simulink model "cvtModel_dashboard_mapped"  (R2023a)
settings: Solver=VariableStepAuto  StartTime=0.0  StopTime=inf  FixedStep=1e-3  RelTol=1e-3  AbsTol=1e-3  EnableMultiTasking=on
PreLoadFcn:
  | m1=3.5;
  | m2=3.2;
  | mr1=0.8;
  | mr2=0.7;
  | speedVector=[1508.85099817596;1518.45723596462;1530.44196592720;1537.65262467286;1544.87011816615;1563.98348990289;1583.08660951818;1616.48460379372;1668.91395283447;1709.42350201510;1752.30812599583;1799.96340381967;1847.59134265301;1904.74008492967;1971.45405650923;2028.61646828115;2083.40038787914;2140.55254752961;2190.54189166781;2259.62068592604;2323.95274795787;2376.37867962481;2443.06531221387;2519.28983511532;2576.50350749443;2612.24923757958;2650.37004246484;2681.37245769738;2717.13869202541;2771.92602899721;2819.56080257817;2855.26894155137;2890.95315890788;2938.61868885316;2976.76341535511;2991.07537688442;3019.63778721441;3045.79436637996;3071.94069342408;3093.34370561560;3114.80823053575;3141.04340929901;3172.04240715774;3186.35436868705;3214.89627477416;3231.51496362732;3267.18209411476;3333.83797033950;3371.93485360807;3421.93444986770;3488.60057821388;3540.98550139507;3586.19052219491;3617.10408570831;3674.22548899447;3712.24719003915;3731.22044944954;3740.69340965949;3759.66325169607;3771.50786933232;3785.72414439486;3792.79810818800;3797.48674505959;3802.17879930499;3806.87085355039;3816.26521416264;3820.89917305322;3827.93896310823;3835.00950952755;3839.71865064202];
  | torqueVector=[15.4893802008608;16.0795925394548;16.6441434720229;17.1317101865136;17.6705997130559;18.1068436154950;18.4661032998565;18.8510243902439;19.0563156384505;19.1846226685796;19.2616068866571;19.3899139167862;19.3129296987087;19.1846226685796;19.3385911047346;19.3129296987087;19.3129296987087;19.2102840746054;18.9793314203730;19.0049928263988;19.1589612625538;19.3385911047346;19.2872682926829;19.3129296987087;19.6721893830703;19.8004964131994;19.8774806312769;20.1597560975610;20.4420315638450;20.4676929698709;20.4420315638450;20.2880631276901;19.9544648493544;20.1597560975610;20.4163701578192;20.5703385939742;20.4163701578192;20.0827718794835;19.6721893830703;19.4155753228120;19.6208665710186;19.8774806312769;20.1340946915351;20.2880631276901;19.9801262553802;19.5695437589670;19.1076384505021;18.8253629842181;18.7227173601148;18.5687489239598;18.3634576757532;18.2351506456241;17.8502295552367;17.4653084648493;17.1317101865136;16.4645136298422;15.8486398852224;15.4380573888092;14.7965222381636;14.3089555236729;13.7444045911047;13.2055150645624;12.6409641319943;12.1020746054519;11.5631850789096;10.5623902439024;9.58725681492108;8.79175322812051;8.22720229555236;7.81661979913916];
  | load Lookuptable_data
model workspace (MAT data in the model file):
  DOWN_TABLE = [0  5  20  35; 0  5  20  35; 0  5  25  40; 0  5  30  50; 0  30  50  80; 0  30  50  80]
  DOWN_TH_BP = [0; 0.05; 0.4; 0.5; 0.9; 1]
  TWAIT = 2
  UP_TABLE = [10  30  50  1000000; 10  30  50  1000000; 15  30  50  1000000; 23  41  60  1000000; 40  70  100  1000000; 40  70  100  1000000]
  UP_TH_BP = [0; 0.25; 0.35; 0.5; 0.9; 1]
  clutchRise = 0.1
  eff_tor_rad = 0.4
  engagement_area = 0.0025
  fric_coeff = 0.5
  num_fric_surf = 6
  p0 = 2000000
  peak_normal = 0.55
  pressThresh = 0.05
  velTol = 0.001
undefined symbols (not defined in the file): vehicle_speed
libraries: fl_lib x22, sdl_lib x9, nesl_utility x8
(part 1 of 2)
CloseFcn:
  | try,close(h1_sdl_car),end
  | clear h1_sdl_car
  | 
  | clear simlog_sdl_car
  | clear logsout_sdl_car
Description:
  | Vehicle with Four-Speed Transmission
  | 
  | Copyright 2008-2016 The MathWorks, Inc.
settings Model: PacingRate=5  Creator=MathWorks
settings SolverCC: AutoScaleAbsTol=off  ZcThreshold=0  ZeroCrossAlgorithm=Adaptive  AlgebraicLoopSolver=TrustRegion
settings DataIOCC: LimitDataPoints=on  MaxDataPoints=10000  SaveOutput=off  DSMLogging=off  SaveTime=off  ReturnWorkspaceOutputs=off  SignalLoggingName=logsout_cvtModel_dashboard
settings OptimizationCC: ExpressionDepthLimit=2147483647  InitFltsAndDblsToZero=on  LifeSpan=inf
settings DebuggingCC: AlgebraicLoopMsg=none  SaveWithParameterizedLinksMsg=none  UnderspecifiedInitializationDetection=Classic  MergeDetectMultiDrivingBlocksExec=none  CheckExecutionContextPreStartOutputMsg=on  SignalResolutionControl=TryResolveAllWithWarning  MaskedZcDiagnostic=none  MultiTaskDSMMsg=warning  MultiTaskCondExecSysMsg=none  SigSpecEnsureSampleTimeMsg=none  FcnCallInpInsideContextMsg=warning  UnconnectedInputMsg=warning  UnconnectedOutputMsg=warning  UnconnectedLineMsg=warning  AllowSymbolicDim=off  StateNameClashWarn=warning  SFUnexpectedBacktrackingDiag=warning  SFNoUnconditionalDefaultTransitionDiag=warning  SFExecutionAtInitializationDiag=none  ArithmeticOperatorsInVariantConditions=warning
settings HardwareCC: ProdBitPerPointer=32  ProdBitPerSizeT=32  ProdBitPerPtrDiffT=32  ProdLargestAtomicFloat=None  ProdIntDivRoundTo=Undefined  ProdEndianess=Unspecified  ProdWordSize=32  ProdHWDeviceType=32-bit Generic  TargetBitPerLong=64  TargetBitPerPointer=64  TargetBitPerSizeT=64  TargetBitPerPtrDiffT=64  TargetLongLongMode=on  TargetIntDivRoundTo=Zero  TargetEndianess=LittleEndian  TargetWordSize=64  TargetHWDeviceType=MATLAB Host  ProdEqTarget=off
settings ModelReferenceCC: UpdateModelReferenceTargets=IfOutOfDate  EnableRefExpFcnMdlSchedulingChecks=on  PropagateSignalLabelsOutOfModel=off
settings SFSimCC: SimUseLocalCustomCode=off  CustomCodeUndefinedFunction=UseInterfaceOnly
settings RTWCC: RTWUseLocalCustomCode=off
settings CodeAppCC: StateflowObjectComments=on
settings GRTTargetCC: TargetLangStandard=C89/C90 (ANSI)  CombineOutputUpdateFcns=off  GRTInterface=on
settings ConfigComp: CovMetricSettings=dw  CovSaveCumulativeToWorkspaceVar=on  CovSaveSingleToWorkspaceVar=on  CovExternalEMLEnable=off  CovBoundaryAbsTol=1.0e-5
settings SimscapeCC: SimscapeNormalizeSystem=off  SimscapeLogType=all  SimscapeLogSimulationStatistics=on

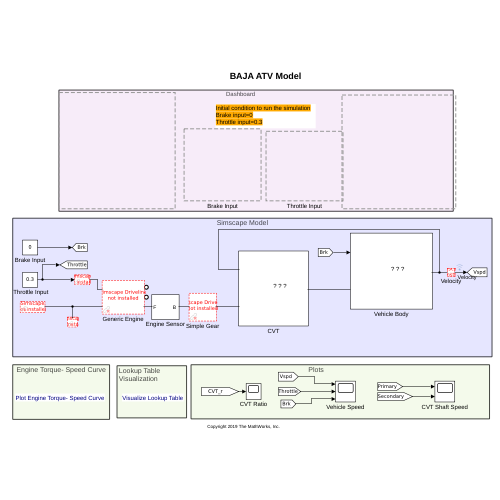
[thumbnail: Simulink's stored preview of the top-level diagram]
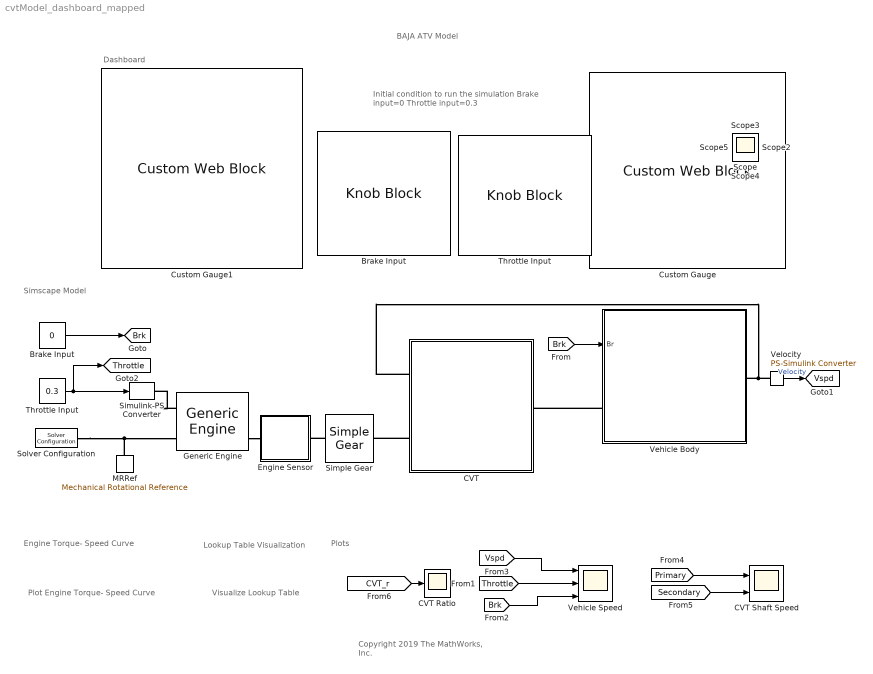
== system cvtModel_dashboard_mapped ==
  note: Initial condition to run the simulation
      | Brake input=0
      | Throttle input=0.3
  note: Dashboard
  note: Simscape Model
  note: Copyright 2019 The MathWorks, Inc.
  note: Plots
  note: Visualize Lookup Table
  note: Lookup Table
      | Visualization
  note: Engine Torque- Speed Curve
  note: Plot Engine Torque- Speed Curve
  note: BAJA ATV Model
  "   Throttle Input " : Constant  Value=0.3
  Brake Input : KnobBlock  LabelPosition=Hide  ScaleMax=0.5  TickInterval=0.10000000000000001
  "Brake Input " : Constant  Value=0
  CVT : Subsystem
      mask Display: image("CVT.jpg")
  CVT Ratio : Scope
  CVT Shaft Speed : Scope  NumInputPorts=2
  Custom Gauge : CustomWebBlock  LabelPosition=Bottom  ShowInitialText=on  Configuration="{\"components\":[{\"name\":\"CircularScaleComponent\",\"settings\":{\"bounds\":{\"max\":100,\"min\":0,\"tickInterval\":\"auto\"},\"direction\":\"cw\",\"flipLimits\":0,\"innerRadius\":0.75,\"internalTickHeightScaleFactor\":1,\"labelColor\":[255,252,199],\"labelFont\":{\"font\":\"Arial\",\"fontSize\":12},\"labelRadius\":0.36,\"labelTransparency\":1,\"minorTickHeightScaleFactor\":0.2,\"needleImage\":{\"size\":[1890,567],\"src\":\"data:image\\/svg+xml;base64,PD94bWwgdmVyc2lvbj0iMS4wIiBlbmNvZGluZz0iVVRGLTgiIHN0YW5kYWxvbmU9Im5vIj8+CjxzdmcKICAgeG1sbnM6ZGM9Imh0dHA6Ly9wdXJsLm9yZy9kYy9lbGVtZW50cy8xLjEvIgogICB4bWxuczpjYz0iaHR0cDovL2NyZWF0aXZlY29tbW9ucy5vcmcvbnMjIgogICB4bWxuczpyZGY9Imh0dHA6Ly93d3cudzMub3JnLzE5OTkvMDIvMjItcmRmLXN5bnRheC1ucyMiCiAgIHhtbG5zOnN2Zz0iaHR0cDovL3d3dy53My5vcmcvMjAwMC9zdmciCiAgIHhtbG5zPSJodHRwOi8vd3d3LnczLm9yZy8yMDAwL3N2ZyIKICAgeG1sbnM6 ...(+4096 chars)\"},\"needleOffset\":[0.14,0],\"needleOrientation\":-45,\"needleRotation\":180,\"needleSize\":{\"height\":0.13,\"width\":0.41},\"outerRadius\":0.9,\"position\":[0.06486742424242424,0.05627705627705628,0.8917748917748918,0.8787878787878788],\"scaleAngle\":270,\"scaleAngleOffset\":135,\"scaleColors\":[],\"scaleColorsSize\":0.2,\"scalePosition\":[0,0,1,1],\"showLabels\":1,\"showMinorTicks\":1,\"showSpanLine\":1,\"showTicks\":1,\"tickColor\":[255,255,200],\"tickTransparency\":1,\"valueBarColor\":[0,114,189],\"valueBarPosition\":[0,0,1,1],\"valueBarSize\":0.2,\"valueBarTransparency\":1}},{\"name\":\"BackgroundImageComponent\",\"settings\":{\"image\":{\"size\":[500,500],\"src\":\"data:image\\/svg+xml;base64,PD94bWwgdmVyc2lvbj0iMS4wIiBlbmNvZGluZz0iVVRGLTgiIHN0YW5kYWxvbmU9Im5vIj8+CjxzdmcKICAgeG1sbnM6ZGM9Imh0dHA6Ly9wdXJsLm9yZy9kYy9lbGVtZW50cy8xLjEvIgogICB4bWxuczpjYz0iaHR0cDovL2NyZWF0aXZlY29tbW9ucy5vcmcvbnMjIgogICB4bWxuczpyZGY9Imh0dHA6Ly93d3cudzMub3JnLzE5OTkvMDIvMjItcmRmLXN5bnRheC1ucyMiCiAgIHhtbG5zOnN2Zz0iaHR0cDovL3d3dy53My5vcmcvMjAwMC9zdmciCiAgIHhtbG5zPSJodHRwOi8vd3d3LnczLm9yZy8yMDAwL3N2ZyIKICAgeG1sbnM6 ...(+9964 chars)\"},\"position\":[0,0,1,1],\"scaleMode\":\"0\"}},{\"name\":\"ForegroundImageComponent\",\"settings\":{\"image\":{\"size\":[0,0],\"src\":\"default\",\"srcOrientation\":[]},\"isForeground\":1,\"position\":[0,0,1,1],\"scaleMode\":\"0\"}}],\"legacySettings\":{\"BackgroundImage\":\"data:image\\/svg+xml;base64,PD94bWwgdmVyc2lvbj0iMS4wIiBlbmNvZGluZz0iVVRGLTgiIHN0YW5kYWxvbmU9Im5vIj8+CjwhLS0gR2VuZXJhdG9yOiBBZG9iZSBJbGx1c3RyYXRvciAxOS4yLjEsIFNWRyBFeHBvcnQgUGx1Zy1JbiAuIFNWRyBWZXJzaW9uOiA2LjAwIEJ1aWxkIDApICAtLT4KCjxzdmcKICAgeG1sbnM6ZGM9Imh0dHA6Ly9wdXJsLm9yZy9kYy9lbGVtZW50cy8xLjEvIgogICB4bWxuczpjYz0iaHR0cDovL2NyZWF0aXZlY29tbW9ucy5vcmcvbnMjIgogICB4bWxuczpyZGY9Imh0dHA6Ly93d3cudzMub3JnLzE5OTkvMDIvMjItcmRmLXN5bnRh ...(+9660 chars)\",\"CenterOffsetX\":\"0\",\"CenterOffsetY\":\"0\",\"GaugeArcColor\":\"#9ec0f7\",\"GaugeArcDefined\":\"true\",\"GaugeArcRadius\":\"0.1358563990074277\",\"GaugeArcRatio\":\"0.8333333333333\",\"GaugeArcRotation\":\"240.5385250290321\",\"GaugeArcStrokeWidth\":\"0.03972965542329953\",\"GaugeArcTransparency\":\"0\",\"GaugeMax\":\"100\",\"GaugeMin\":\"0\",\"GaugeTickColor\":\"#faf5c8\",\"GaugeTickTransparency\":\"1\",\"GaugeTickVisible\":\"true\",\"GaugeValue\":\"0\",\"NeedleHeight\":\"0.11602152693163792\",\"NeedleImage\":\"data:image\\/svg+xml;base64,PD94bWwgdmVyc2lvbj0iMS4wIiBlbmNvZGluZz0idXRmLTgiPz4KPCEtLSBHZW5lcmF0b3I6IEFkb2JlIElsbHVzdHJhdG9yIDE5LjIuMSwgU1ZHIEV4cG9ydCBQbHVnLUluIC4gU1ZHIFZlcnNpb246IDYuMDAgQnVpbGQgMCkgIC0tPgo8c3ZnIHZlcnNpb249IjEuMSIgeG1sbnM9Imh0dHA6Ly93d3cudzMub3JnLzIwMDAvc3ZnIiB4bWxuczp4bGluaz0iaHR0cDovL3d3dy53My5vcmcvMTk5OS94bGluayIgeD0iMHB4IiB5PSIwcHgiCgkgdmlld0JveD0iMCAwIDIwMCA1MCIgc3R5bGU9ImVuYWJsZS1iYWNrZ3JvdW5kOm5ldyAw ...(+9940 chars)\",\"NeedleInitialRotation\":\"-59.94322499147643\",\"NeedleWidth\":\"0.1911368983686954\",\"NeedleXPos\":\"0.3802298124325669\",\"NeedleYPos\":\"0.48117305677424654\",\"ScaleColorsJSON\":\"{\\\"Min\\\":0,\\\"Max\\\":0,\\\"Color\\\":[0,0.44705882352941173,0.74117647058823533]}\",\"ValueArcColor\":\"#1759b0\",\"ValueArcTransparency\":\"1\"},\"settings\":{\"BindingType\":\"signal\",\"backgroundOffset\":0.14,\"backgroundOpacity\":1,\"fixedAspectRatio\":\"on\",\"showBackgroundColor\":0,\"version\":\"R2023a\"},\"type\":\"CircularGauge\"}"
  Custom Gauge1 : CustomWebBlock  LabelPosition=Bottom  ShowInitialText=on  Configuration="{\"components\":[{\"name\":\"CircularScaleComponent\",\"settings\":{\"bounds\":{\"max\":100,\"min\":0,\"tickInterval\":\"auto\"},\"direction\":\"cw\",\"flipLimits\":0,\"innerRadius\":0.75,\"internalTickHeightScaleFactor\":1,\"labelColor\":[255,252,199],\"labelFont\":{\"font\":\"Arial\",\"fontSize\":12},\"labelRadius\":0.36,\"labelTransparency\":1,\"minorTickHeightScaleFactor\":0.2,\"needleImage\":{\"size\":[1890,567],\"src\":\"data:image\\/svg+xml;base64,PD94bWwgdmVyc2lvbj0iMS4wIiBlbmNvZGluZz0iVVRGLTgiIHN0YW5kYWxvbmU9Im5vIj8+CjxzdmcKICAgeG1sbnM6ZGM9Imh0dHA6Ly9wdXJsLm9yZy9kYy9lbGVtZW50cy8xLjEvIgogICB4bWxuczpjYz0iaHR0cDovL2NyZWF0aXZlY29tbW9ucy5vcmcvbnMjIgogICB4bWxuczpyZGY9Imh0dHA6Ly93d3cudzMub3JnLzE5OTkvMDIvMjItcmRmLXN5bnRheC1ucyMiCiAgIHhtbG5zOnN2Zz0iaHR0cDovL3d3dy53My5vcmcvMjAwMC9zdmciCiAgIHhtbG5zPSJodHRwOi8vd3d3LnczLm9yZy8yMDAwL3N2ZyIKICAgeG1sbnM6 ...(+4096 chars)\"},\"needleOffset\":[0.14,0],\"needleOrientation\":-45,\"needleRotation\":180,\"needleSize\":{\"height\":0.13,\"width\":0.41},\"outerRadius\":0.9,\"position\":[0.06486742424242424,0.05627705627705628,0.8917748917748918,0.8787878787878788],\"scaleAngle\":270,\"scaleAngleOffset\":135,\"scaleColors\":[],\"scaleColorsSize\":0.2,\"scalePosition\":[0,0,1,1],\"showLabels\":1,\"showMinorTicks\":1,\"showSpanLine\":1,\"showTicks\":1,\"tickColor\":[255,255,200],\"tickTransparency\":1,\"valueBarColor\":[0,114,189],\"valueBarPosition\":[0,0,1,1],\"valueBarSize\":0.2,\"valueBarTransparency\":1}},{\"name\":\"BackgroundImageComponent\",\"settings\":{\"image\":{\"size\":[500,500],\"src\":\"data:image\\/svg+xml;base64,PD94bWwgdmVyc2lvbj0iMS4wIiBlbmNvZGluZz0iVVRGLTgiIHN0YW5kYWxvbmU9Im5vIj8+CjxzdmcKICAgeG1sbnM6ZGM9Imh0dHA6Ly9wdXJsLm9yZy9kYy9lbGVtZW50cy8xLjEvIgogICB4bWxuczpjYz0iaHR0cDovL2NyZWF0aXZlY29tbW9ucy5vcmcvbnMjIgogICB4bWxuczpyZGY9Imh0dHA6Ly93d3cudzMub3JnLzE5OTkvMDIvMjItcmRmLXN5bnRheC1ucyMiCiAgIHhtbG5zOnN2Zz0iaHR0cDovL3d3dy53My5vcmcvMjAwMC9zdmciCiAgIHhtbG5zPSJodHRwOi8vd3d3LnczLm9yZy8yMDAwL3N2ZyIKICAgeG1sbnM6 ...(+9964 chars)\"},\"position\":[0,0,1,1],\"scaleMode\":\"0\"}},{\"name\":\"ForegroundImageComponent\",\"settings\":{\"image\":{\"size\":[0,0],\"src\":\"default\",\"srcOrientation\":[]},\"isForeground\":1,\"position\":[0,0,1,1],\"scaleMode\":\"0\"}}],\"legacySettings\":{\"BackgroundImage\":\"data:image\\/svg+xml;base64,PD94bWwgdmVyc2lvbj0iMS4wIiBlbmNvZGluZz0iVVRGLTgiIHN0YW5kYWxvbmU9Im5vIj8+CjwhLS0gR2VuZXJhdG9yOiBBZG9iZSBJbGx1c3RyYXRvciAxOS4yLjEsIFNWRyBFeHBvcnQgUGx1Zy1JbiAuIFNWRyBWZXJzaW9uOiA2LjAwIEJ1aWxkIDApICAtLT4KCjxzdmcKICAgeG1sbnM6ZGM9Imh0dHA6Ly9wdXJsLm9yZy9kYy9lbGVtZW50cy8xLjEvIgogICB4bWxuczpjYz0iaHR0cDovL2NyZWF0aXZlY29tbW9ucy5vcmcvbnMjIgogICB4bWxuczpyZGY9Imh0dHA6Ly93d3cudzMub3JnLzE5OTkvMDIvMjItcmRmLXN5bnRh ...(+9660 chars)\",\"CenterOffsetX\":\"0\",\"CenterOffsetY\":\"0\",\"GaugeArcColor\":\"#9ec0f7\",\"GaugeArcDefined\":\"true\",\"GaugeArcRadius\":\"0.1358563990074277\",\"GaugeArcRatio\":\"0.8333333333333\",\"GaugeArcRotation\":\"240.5385250290321\",\"GaugeArcStrokeWidth\":\"0.03972965542329953\",\"GaugeArcTransparency\":\"0\",\"GaugeMax\":\"10000\",\"GaugeMin\":\"0\",\"GaugeTickColor\":\"#faf5c8\",\"GaugeTickTransparency\":\"1\",\"GaugeTickVisible\":\"true\",\"GaugeValue\":\"0\",\"NeedleHeight\":\"0.11602152693163792\",\"NeedleImage\":\"data:image\\/svg+xml;base64,PD94bWwgdmVyc2lvbj0iMS4wIiBlbmNvZGluZz0idXRmLTgiPz4KPCEtLSBHZW5lcmF0b3I6IEFkb2JlIElsbHVzdHJhdG9yIDE5LjIuMSwgU1ZHIEV4cG9ydCBQbHVnLUluIC4gU1ZHIFZlcnNpb246IDYuMDAgQnVpbGQgMCkgIC0tPgo8c3ZnIHZlcnNpb249IjEuMSIgeG1sbnM9Imh0dHA6Ly93d3cudzMub3JnLzIwMDAvc3ZnIiB4bWxuczp4bGluaz0iaHR0cDovL3d3dy53My5vcmcvMTk5OS94bGluayIgeD0iMHB4IiB5PSIwcHgiCgkgdmlld0JveD0iMCAwIDIwMCA1MCIgc3R5bGU9ImVuYWJsZS1iYWNrZ3JvdW5kOm5ldyAw ...(+9940 chars)\",\"NeedleInitialRotation\":\"-59.94322499147643\",\"NeedleWidth\":\"0.1911368983686954\",\"NeedleXPos\":\"0.3802298124325669\",\"NeedleYPos\":\"0.48117305677424654\",\"ScaleColorsJSON\":\"{\\\"Min\\\":0,\\\"Max\\\":0,\\\"Color\\\":[0.92941176470588238,0.69411764705882351,0.12549019607843137]}\",\"ValueArcColor\":\"#1759b0\",\"ValueArcTransparency\":\"1\"},\"settings\":{\"BindingType\":\"signal\",\"backgroundOffset\":0.14,\"backgroundOpacity\":1,\"fixedAspectRatio\":\"on\",\"showBackgroundColor\":0,\"version\":\"R2023a\"},\"type\":\"CircularGauge\"}"
  Engine Sensor : Subsystem
  Generic Engine : sdl_lib/Engines/Generic Engine  model_parameterization=2  engine_type=1  P_max=100 kW  w_P_max=4500 rpm  w_max=5000 rpm  w_min=500 rpm  w_tab=speedVector rpm  trq_tab=torqueVector N*m  pwr_tab=[20, 40, 78, 120, 145, 148, 125, 60] kW  interp_method=simscape.enum.interpolation.linear  model_inertia=1  inertia=1 kg*m^2  initial_velocity=2100 rpm  model_time_constant=0  time_constant=0.4 s  T0=0  w_thr=100 rpm  idle_speed=0  idle_speed_reference=2500 rpm  tau_controller=1 s  idle_w_thr=1 rpm  redline=0  redline_speed=5000 rpm  tau_redline=1 s  redline_w_thr=1 rpm  fc_model=0  fc_per_rev=25 mg/rev  displaced_volume=400 cm^3  rev_per_cycle=2  fc_w_tab=[1000, 2000, 3000, 4000, 5000, 6000] rpm  fc_trq_tab=[0, 80, 160, 200, 240, 320, 360, 400] N*m  fc_tab=[.5, .9, 1.4, 1.6, 1.9, 2.7, 3.4, 4.4; 1, 1.7, 2.7, 3.1, 3.6, 5, 6, 7.4; 1.4, 2.7, 4, 4.8, 5.6, 7.5, 8.5, 10.5; 2, 3.6, 5.8, 6.7, 8, 10.4, 11.7, 13.3; 2.5, 4.8, 7.9, 9.4, 10.8, 14, 16.2, 18.6; 3.1, 6, 10.3, 11.9, 13.8, 18.4, 22, 26.5] g/s  bmep_tab=[0, 250, 500, 625, 750, 1000, 1150, 1250] kPa  bsfc_tab=[410, 380, 300, 280, 270, 290, 320, 380; 410, 370, 290, 270, 260, 270, 285, 320; 415, 380, 290, 275, 265, 270, 270, 300; 420, 390, 310, 290, 285, 280, 280, 285; 430, 410, 340, 320, 310, 300, 310, 320; 450, 430, 370, 340, 330, 330, 350, 380] g/hr/kW  fc_interp_method=simscape.enum.interpolation.linear
      settings: SourceProductName=Simscape Driveline
  MRRef : fl_lib/Mechanical/Rotational Elements/Mechanical Rotational Reference
  Simple Gear : sdl_lib/Gears/Simple Gear  ratio=4  rotation_direction=1  friction_model=1  T_noload=0.1 N*m  T_nom=5 N*m  efficiency_nom=0.8  efficiency=0.8  mu_visc=[0, 0] N*m/(rad/s)  w_thr=0.01 rad/s  pwr_thr=0.001 W  enable_faults=0  efficiency_fault=0.05  external_fault=simscape.enum.onoff.off  temporal_fault=0  fault_time=5 s  fault_angles=pi / 12 rad  report_fault=1  temperature_TLU=[280, 300, 320] K  load_TLU=[1, 5, 10] N*m  efficiency_TLU=[.95, .9, .85]  efficiency_TLU2=[.85, .8, .75; .95, .9, .85; .85, .8, .7]  thermal_mass=50 J/K  T_init=300 K
      settings: SourceProductName=Simscape Driveline
  Simulink-PS Converter : nesl_utility/Simulink-PS Converter  PhysicalDomain=network_engine_domain  SubClassName=ps_input  LeftPortType=input  RightPortType=output  PseudoPeriodic=off  Frequencies=[]  NoiseDistribution=none  NoiseParameters=[]  Unit=1  AffineConversion=off  FilteringAndDerivatives=zero  SimscapeFilterOrder=1  InputFilterTimeConstant=0.001  UdotUserProvided=1
  Solver Configuration : nesl_utility/Solver Configuration  PhysicalDomain=network_engine_domain  SubClassName=solver  LeftPortType=input  RightPortType=generic  Tones=[]  Harmonics=[]  SimulateNoise=off  Profile=off  UseLocalSampling=off  EnableSwitchedLinearOptims=on  FrequencyDomain=off  UseCCode=off  RelTol=0.001  AbsTol=1e-06  MinStep=1e-09  ToWorkspace=off  RevertToSquareIcSolve=off  NumHomotopyIterations=100  PhasorMode=off  PhasorModeNumHarmonics=1  DoDC=off  ResidualTolerance=1e-9  UseLocalSolver=off  LocalSolverChoice=NE_BACKWARD_EULER_ADVANCER  LocalSolverSampleTime=0.001  DoFixedCost=off  MaxNonlinIter=3  MaxModeIter=2  LinearAlgebra=Sparse  EquationFormulation=NE_TIME_EF  DelaysMemoryBudget=1024  AutomaticFiltering=on  FilteringTimeConstant=0.001  PartitionStorageMethod=AS_NEEDED  PartitionMemoryBudget=1024
  Throttle Input : KnobBlock  LabelPosition=Hide  ScaleMin=0.29999999999999999  ScaleMax=1  TickInterval=0.10000000000000001
  Vehicle Body : Subsystem  Tag=PublishSubsystem
      mask Display: image("vehicleBody.jpg")
  Vehicle Speed : Scope  NumInputPorts=3
  Velocity : nesl_utility/PS-Simulink Converter  PhysicalDomain=network_engine_domain  SubClassName=ps_output  LeftPortType=input  RightPortType=output  PseudoPeriodic=off  Frequencies=[]  Unit=km/hr  AffineConversion=off
  Scope{,2..5} (5 alike) : Scope
  tag scope: Brk=global, Throttle=global, Vspd=global
  wires:
  "   Throttle Input "/1 -> Simulink-PS Converter/1, [Throttle]
  [Brk] -> Vehicle Body/1(Br)
  "Brake Input "/1 -> [Brk]
  [CVT_r] -> CVT Ratio/1
  [Primary] -> CVT Shaft Speed/1
  [Vspd] -> Vehicle Speed/1
  [Secondary] -> CVT Shaft Speed/2
  [Brk] -> Vehicle Speed/3
  [Throttle] -> Vehicle Speed/2
  Velocity/1 -> [Vspd]  "Velocity"
  connections:
  Generic Engine/LConn1 -- Simulink-PS Converter/RConn1
  MRRef/LConn1 -- Solver Configuration/RConn1 -- Generic Engine/LConn2
  Generic Engine/RConn3 -- Engine Sensor/LConn1
  Simple Gear/LConn1 -- Engine Sensor/RConn1
  CVT/LConn2 -- Simple Gear/RConn1
  Vehicle Body/LConn1 -- CVT/RConn1
  Velocity/LConn1 -- CVT/LConn1 -- Vehicle Body/RConn1
